simulink model "tether005_th"  (R2022a)
settings: Solver=ode23s  StartTime=0.0  StopTime=simTime  MaxStep=0.01  RelTol=1e-3
values from neighbouring files (symbols this model uses):
  linkFlowVelVecs = [10*ones(1,numNodes-1);10*ones(1,numNodes-1);.001*ones(1,numNodes-1)]    [tether005_ts.m]
  OriginalLengths = [((TetherLength-TopLinkLength)/(numNodes-2))*ones(1,numNodes-2),TopLinkLength]    [tether005_ts.m]
  ReelInVel = -(LengthI-LengthF)/simTime    (= -3.99)    [tether005_ts.m]
  TetherLength = 400    [tether005_ts.m]
libraries: tether005_ul x1
settings Model: Creator=mitch  LastModifiedBy=lhill8
settings SolverCC: AlgebraicLoopSolver=TrustRegion
settings DebuggingCC: UnconnectedInputMsg=warning  UnconnectedOutputMsg=warning  UnconnectedLineMsg=warning  SFMachineParentedDataDiag=warning

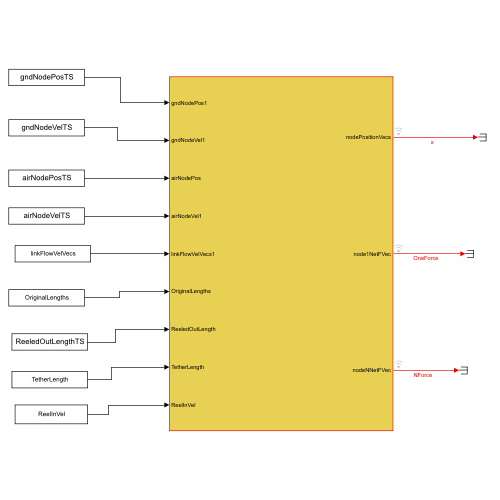
[thumbnail: Simulink's stored preview of the top-level diagram]
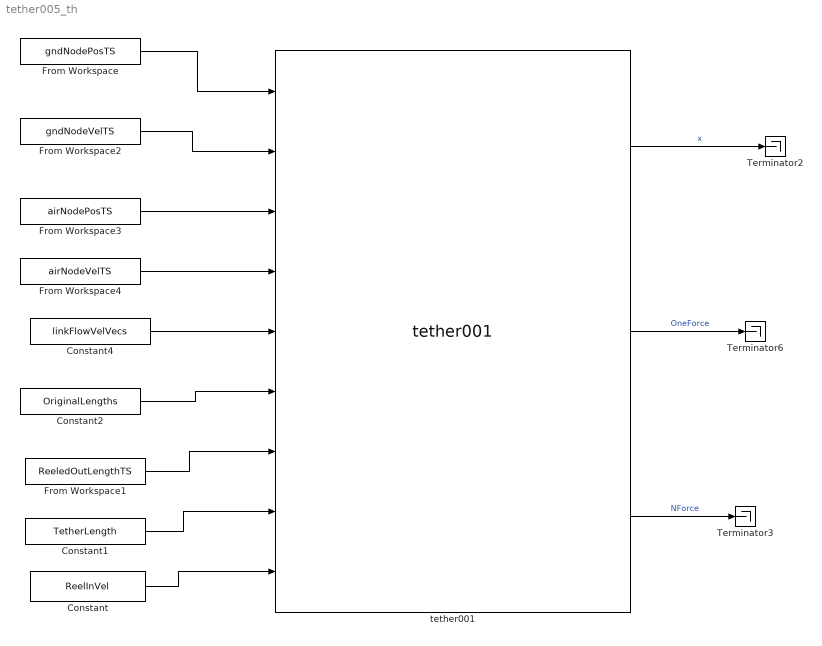
== system tether005_th ==
  Constant : Constant  Value=ReelInVel
  Constant1 : Constant  Value=TetherLength
  Constant2 : Constant  Value=OriginalLengths
  Constant4 : Constant  Value=linkFlowVelVecs
  From Workspace : FromWorkspace  VariableName=gndNodePosTS
  From Workspace1 : FromWorkspace  VariableName=ReeledOutLengthTS  Interpolate=off  OutputAfterFinalValue=Holding final value
  From Workspace2 : FromWorkspace  VariableName=gndNodeVelTS
  From Workspace3 : FromWorkspace  VariableName=airNodePosTS
  From Workspace4 : FromWorkspace  VariableName=airNodeVelTS
  Terminator2 : Terminator
  Terminator3 : Terminator
  Terminator6 : Terminator
  tether001 : tether005_ul/tether001  SystemSampleTime=-1  VariantActivationTime=update diagram  Latency=0  AutoFrameSizeCalculation=off
  wires:
  From Workspace/1 -> tether001/1
  From Workspace2/1 -> tether001/2
  From Workspace3/1 -> tether001/3
  From Workspace4/1 -> tether001/4
  Constant4/1 -> tether001/5
  Constant2/1 -> tether001/6
  From Workspace1/1 -> tether001/7
  Constant1/1 -> tether001/8
  Constant/1 -> tether001/9
  tether001/3 -> Terminator3/1  "NForce"
  tether001/2 -> Terminator6/1  "OneForce"
  tether001/1 -> Terminator2/1  "x"
